simulink model "b2b_th1"  (R2018a)
settings: Solver=VariableStepAuto  StartTime=0.0  StopTime=100  RelTol=1e-3
libraries: simulink x2
settings Model: Creator=Huy  LastModifiedBy=Huy

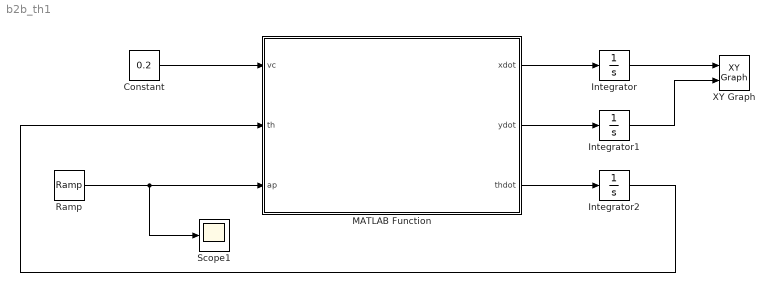
== system b2b_th1 ==
  Constant : Constant  Value=0.2
  Integrator : Integrator
  Integrator1 : Integrator
  Integrator2 : Integrator
  MATLAB Function : MATLAB Function  TreatAsAtomicUnit=on
  Ramp : simulink/Sources/Ramp  slope=0.5  start=0.5  InitialOutput=0
  Scope1 : Scope
  XY Graph : simulink/Sinks/XY Graph  xmin=-0.5  xmax=0.5  ymin=-1  ymax=0.5  st=1
  wires:
  MATLAB Function/1(xdot) -> Integrator/1
  Constant/1 -> MATLAB Function/1(vc)
  MATLAB Function/2(ydot) -> Integrator1/1
  MATLAB Function/3(thdot) -> Integrator2/1
  Integrator/1 -> XY Graph/1
  Integrator1/1 -> XY Graph/2
  Ramp/1 -> Scope1/1, MATLAB Function/3(ap)
  Integrator2/1 -> MATLAB Function/2(th)

== matlab function b2b_th1/MATLAB Function ==
  data: vc input; xdot output; th input; ap input; ydot output; thdot output
function [xdot,ydot,thdot] = tricycle (vc,th,ap)
 %TH1: banh truoc dieu huong va dieu khien toc do
 % ap = alpha
 vmax = 0.36; % van toc cuc dai cua robot
 amax = 0.28; % gia toc cuc dai cua robot
 apmax = (pi/4)*180/pi; % goc lai cuc dai cua robot = 45 do
 wmax = 0.30; % van toc goc cuc dai cua robot
 G = 13; %Nhom
 d = sqrt(2.5 + 0.1*G); % chieu dai co so
 xdot = vc*cos(th)*cos(ap);
 ydot = vc*sin(th)*cos(ap);
 thdot = (vc/d)*sin(ap);
